simulink model "add_entry_model_tester_2"  (R2020b)
settings: Solver=FixedStepDiscrete  StartTime=0.0  StopTime=24  FixedStep=0.1  RelTol=1e-3
undefined symbols (not defined in the file or in its folder): test_input
libraries: simulink x2
settings Model: Creator=rsub  LastModifiedBy=rsub

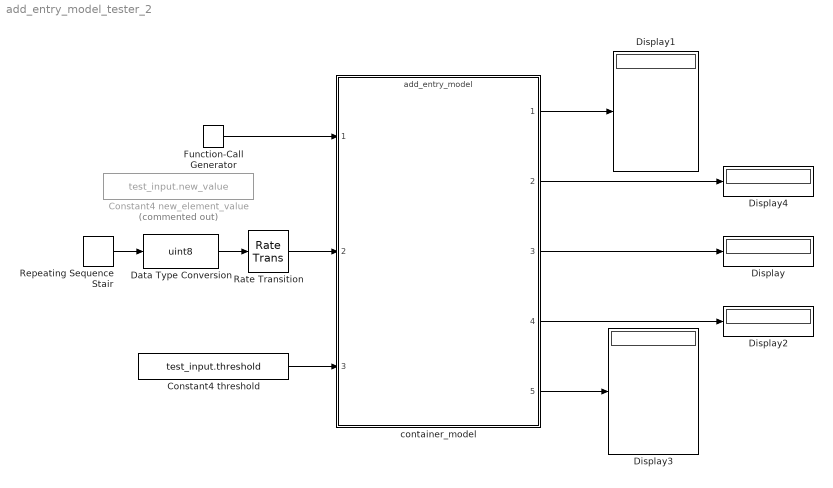
== system add_entry_model_tester_2 ==
  Constant4 new_element_value : Constant  Commented=on  Value=test_input.new_value
  Constant4 threshold : Constant  Value=test_input.threshold
  Data Type Conversion : DataTypeConversion  OutDataTypeStr=uint8
  Display{,1..4} (5 alike) : Display
  Function-Call Generator : simulink/Ports & Subsystems/Function-Call Generator  sample_time=5  numberOfIterations=1  DisallowWideOutput=off
  Rate Transition : RateTransition  Integrity=off  Deterministic=off  OutPortSampleTime=5
  Repeating Sequence Stair : simulink/Sources/Repeating Sequence Stair  OutValues=[10 11 12 13 14 15].'  tsamp=5  OutMin=[]  OutMax=[]  OutDataTypeStr=double  OutputDataTypeScalingMode=double  OutDataType=fixdt(0,8)  ConRadixGroup=Best Precision: Vector-wise  OutScaling=2^-12
  container_model : ModelReference  ModelNameDialog=add_entry_model.slx  ScheduleRates=on  ModelReferenceVersion=1.281
  wires:
  container_model/1 -> Display1/1
  container_model/4 -> Display2/1
  container_model/3 -> Display/1
  container_model/2 -> Display4/1
  Rate Transition/1 -> container_model/2
  Constant4 threshold/1 -> container_model/3
  container_model/5 -> Display3/1
  Repeating Sequence Stair/1 -> Data Type Conversion/1
  Data Type Conversion/1 -> Rate Transition/1
  Function-Call Generator/1 -> container_model/1
